simulink model "BSSLab1"  (R2024b)
settings: Solver=VariableStepAuto  StartTime=0.0  StopTime=10.0  RelTol=1e-3
settings Model: Creator=jaimiem  LastModifiedBy=jaimiem

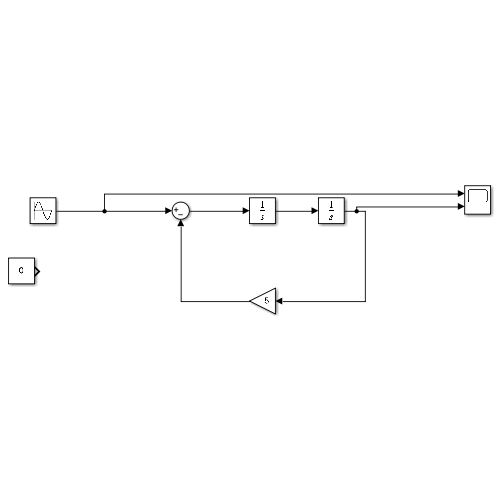
[thumbnail: Simulink's stored preview of the top-level diagram]
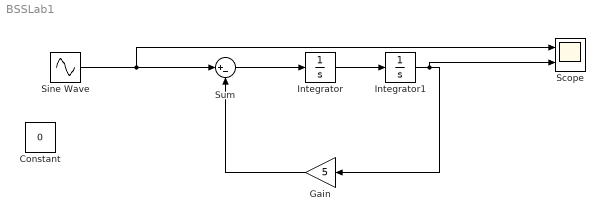
== system BSSLab1 ==
  Constant : Constant  Value=0
  Gain : Gain  Gain=5
  Integrator : Integrator
  Integrator1 : Integrator  InitialCondition=-5
  Scope : Scope  NumInputPorts=2
  Sine Wave : Sin  Frequency=sqrt(5)  Phase=sqrt(5)  SampleTime=0
  Sum : Sum  Inputs=|+-
  wires:
  Integrator/1 -> Integrator1/1
  Integrator1/1 -> Scope/2, Gain/1
  Sum/1 -> Integrator/1
  Gain/1 -> Sum/2
  Sine Wave/1 -> Scope/1, Sum/1
